simulink model "Rull_tunet_vs_ikketunet"  (R2022a)
settings: Solver=VariableStepAuto  StartTime=0.0  StopTime=25  RelTol=1e-3
values from neighbouring files (symbols this model uses):
  B_r_t = 0.000799434    [Modell_verdier.m]
  C_D = 1.28    [Modell_verdier.m]
  Fb = 226    [Modell_verdier.m]
  g = 9.81    [Modell_verdier.m]
  I_rull = 1.28294    [Modell_verdier.m]
  phi_motor_rull = deg2rad(90-61.7)    [Modell_verdier.m]
  r_Fb = 0.036    [Modell_verdier.m]
  r_motor_rull = 0.277    [Modell_verdier.m]
  tetthet_vann = 1000    [Modell_verdier.m]
libraries: simulink_extras x8, spsFirstOrderFilterLib x2
settings Model: Creator=andre  LastModifiedBy=andre

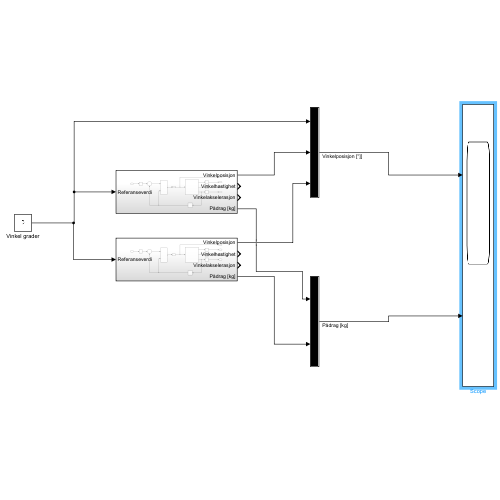
[thumbnail: Simulink's stored preview of the top-level diagram]
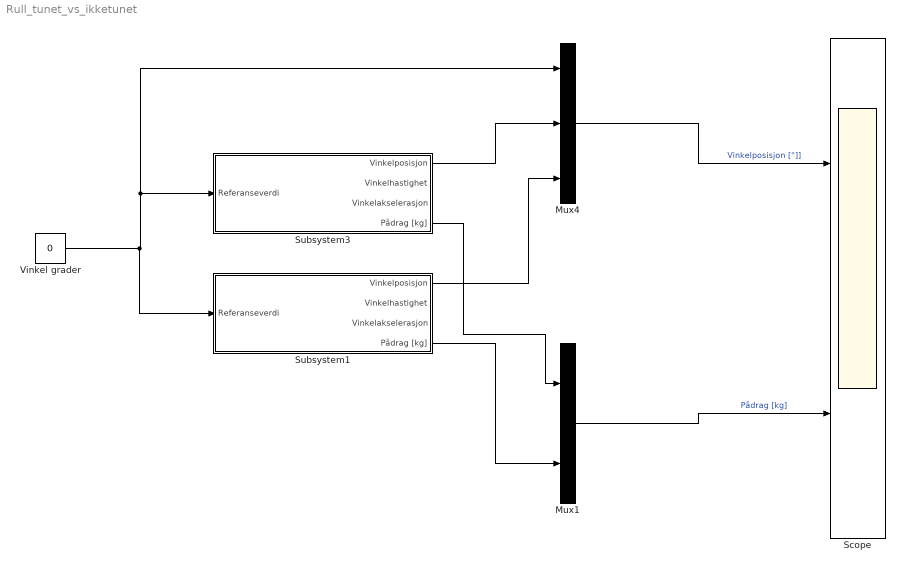
== system Rull_tunet_vs_ikketunet ==
  Mux1 : Mux  Inputs=2
  Mux4 : Mux  Inputs=3
  Scope : Scope  NumInputPorts=2
  Subsystem1 : Subsystem
  Subsystem3 : Subsystem
  Vinkel grader : Constant  Value=0
  wires:
  Vinkel grader/1 -> Subsystem1/1(Referanseverdi), Mux4/1, Subsystem3/1(Referanseverdi)
  Subsystem3/1(Vinkelposisjon) -> Mux4/2
  Subsystem1/1(Vinkelposisjon) -> Mux4/3
  Subsystem1/4(Pådrag [kg]) -> Mux1/2
  Subsystem3/4(Pådrag [kg]) -> Mux1/1
  Mux4/1 -> Scope/1  "Vinkelposisjon [°]]"
  Mux1/1 -> Scope/2  "Pådrag [kg]"

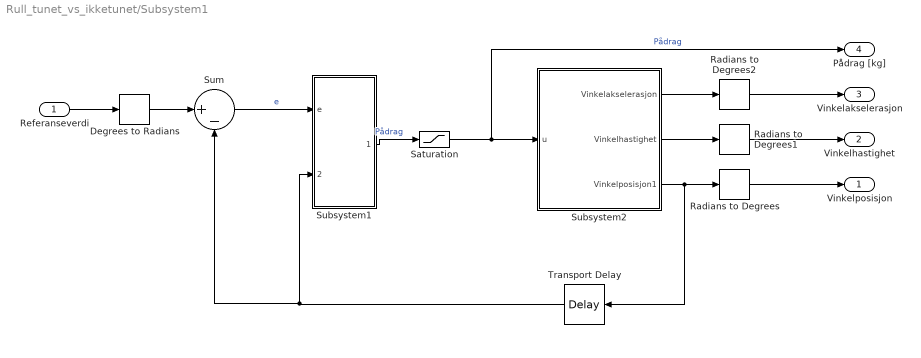
== system Rull_tunet_vs_ikketunet/Subsystem1 ==
  Referanseverdi : Inport
  Degrees to Radians : simulink_extras/Transformations/Degrees to Radians
  Radians to Degrees : simulink_extras/Transformations/Radians to Degrees
  Radians to Degrees1 : simulink_extras/Transformations/Radians to Degrees
  Radians to Degrees2 : simulink_extras/Transformations/Radians to Degrees
  Saturation : Saturate  UpperLimit=2.8  LowerLimit=-2.8
  Subsystem1 : Subsystem
  Subsystem2 : Subsystem
  Sum : Sum  Inputs=|+-
  Transport Delay : TransportDelay  DelayTime=0.2
  Vinkelposisjon : Outport
  Vinkelhastighet : Outport  Port=2
  Vinkelakselerasjon : Outport  Port=3
  Pådrag [kg] : Outport  Port=4
  wires:
  Subsystem2/1(" Vinkelakselerasjon") -> Radians to Degrees2/1
  Sum/1 -> Subsystem1/1(e)  "e"
  Subsystem2/3(Vinkelposisjon1) -> Transport Delay/1, Radians to Degrees/1
  Radians to Degrees/1 -> Vinkelposisjon/1
  Referanseverdi/1 -> Degrees to Radians/1
  Transport Delay/1 -> Sum/2, Subsystem1/2(y_sensor)
  Degrees to Radians/1 -> Sum/1
  Radians to Degrees1/1 -> Vinkelhastighet/1
  Subsystem2/2(" Vinkelhastighet") -> Radians to Degrees1/1
  Saturation/1 -> Pådrag [kg]/1, Subsystem2/1(u)  "Pådrag"
  Subsystem1/1(Pådrag) -> Saturation/1  "Pådrag"
  Radians to Degrees2/1 -> Vinkelakselerasjon/1

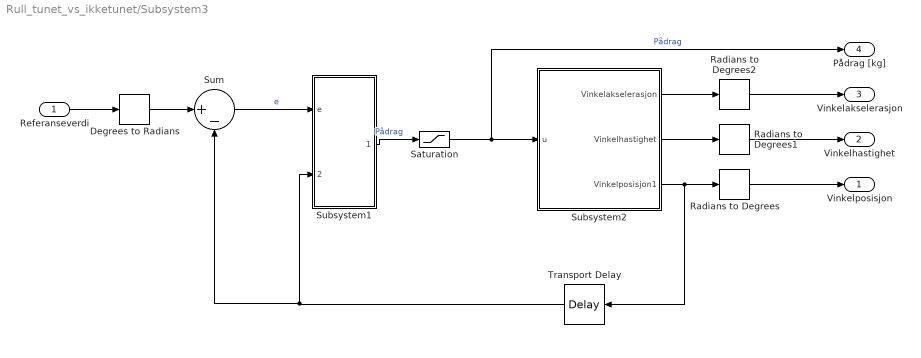
== system Rull_tunet_vs_ikketunet/Subsystem3 ==
  Referanseverdi : Inport
  Degrees to Radians : simulink_extras/Transformations/Degrees to Radians
  Radians to Degrees : simulink_extras/Transformations/Radians to Degrees
  Radians to Degrees1 : simulink_extras/Transformations/Radians to Degrees
  Radians to Degrees2 : simulink_extras/Transformations/Radians to Degrees
  Saturation : Saturate  UpperLimit=2.8  LowerLimit=-2.8
  Subsystem1 : Subsystem
  Subsystem2 : Subsystem
  Sum : Sum  Inputs=|+-
  Transport Delay : TransportDelay  DelayTime=0.2
  Vinkelposisjon : Outport
  Vinkelhastighet : Outport  Port=2
  Vinkelakselerasjon : Outport  Port=3
  Pådrag [kg] : Outport  Port=4
  wires:
  Subsystem2/1(" Vinkelakselerasjon") -> Radians to Degrees2/1
  Sum/1 -> Subsystem1/1(e)  "e"
  Subsystem2/3(Vinkelposisjon1) -> Transport Delay/1, Radians to Degrees/1
  Radians to Degrees/1 -> Vinkelposisjon/1
  Referanseverdi/1 -> Degrees to Radians/1
  Transport Delay/1 -> Sum/2, Subsystem1/2(y_sensor)
  Degrees to Radians/1 -> Sum/1
  Radians to Degrees1/1 -> Vinkelhastighet/1
  Subsystem2/2(" Vinkelhastighet") -> Radians to Degrees1/1
  Saturation/1 -> Pådrag [kg]/1, Subsystem2/1(u)  "Pådrag"
  Subsystem1/1(Pådrag) -> Saturation/1  "Pådrag"
  Radians to Degrees2/1 -> Vinkelakselerasjon/1

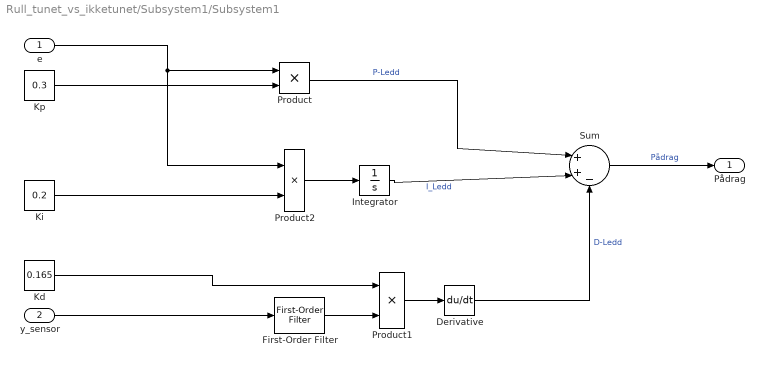
== system Rull_tunet_vs_ikketunet/Subsystem1/Subsystem1 ==
  e : Inport
  y_sensor : Inport  Port=2
  Derivative : Derivative
  First-Order Filter : spsFirstOrderFilterLib/First-Order Filter  FilterType=Lowpass  Tc=(1.5/3.8)*0.05  Ts=0  Initialize=on  Vac_Init=[0, 0, 60]  Vdc_Init=0  PlotResponse=off  FreqRange="[0,  200,  1]"
  Integrator : Integrator  LimitOutput=on  UpperSaturationLimit=0.3  LowerSaturationLimit=-0.3
  Kd : Constant  Value=0.165
  Ki : Constant  Value=0.2
  Kp : Constant  Value=0.3
  Product : Product
  Product1 : Product
  Product2 : Product
  Sum : Sum  Inputs=|++-
  Pådrag : Outport
  wires:
  Product2/1 -> Integrator/1
  Kp/1 -> Product/2
  Product/1 -> Sum/1  "P-Ledd"
  y_sensor/1 -> First-Order Filter/1
  Kd/1 -> Product1/1
  e/1 -> Product/1, Product2/1
  Ki/1 -> Product2/2
  First-Order Filter/1 -> Product1/2
  Integrator/1 -> Sum/2  "I_Ledd"
  Sum/1 -> Pådrag/1  "Pådrag"
  Product1/1 -> Derivative/1
  Derivative/1 -> Sum/3  "D-Ledd"

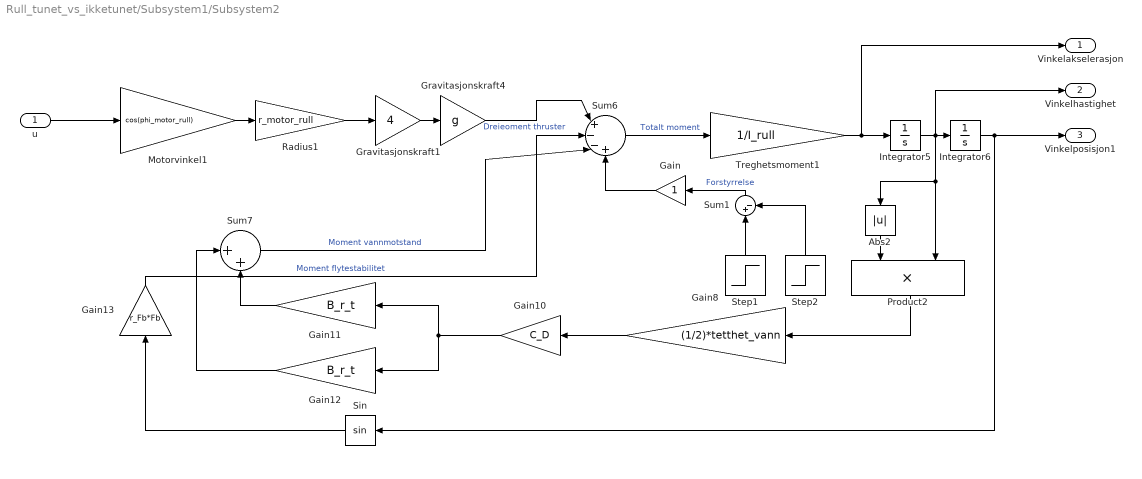
== system Rull_tunet_vs_ikketunet/Subsystem1/Subsystem2 ==
  u : Inport
  Abs2 : Abs  SaturateOnIntegerOverflow=off
  Gain : Gain
  Gain10 : Gain  Gain=C_D
  Gain11 : Gain  Gain=B_r_t
  Gain12 : Gain  Gain=B_r_t
  Gain13 : Gain  Gain=r_Fb*Fb
  Gain8 : Gain  Gain=(1/2)*tetthet_vann
  Gravitasjonskraft1 : Gain  Gain=4
  Gravitasjonskraft4 : Gain  Gain=g
  Integrator5 : Integrator
  Integrator6 : Integrator
  Motorvinkel1 : Gain  Gain=cos(phi_motor_rull)
  Product2 : Product
  Radius1 : Gain  Gain=r_motor_rull
  Sin : Trigonometry
  Step1 : Step  Time=7  After=5  SampleTime=0
  Step2 : Step  Time=10  After=0  SampleTime=0
  Sum1 : Sum  Inputs=|+-
  Sum6 : Sum  Inputs=|+--+
  Sum7 : Sum  Inputs=|++
  Treghetsmoment1 : Gain  Gain=1/I_rull
  " Vinkelakselerasjon" : Outport
  " Vinkelhastighet" : Outport  Port=2
  Vinkelposisjon1 : Outport  Port=3
  wires:
  Integrator6/1 -> Vinkelposisjon1/1, Sin/1
  Motorvinkel1/1 -> Radius1/1
  Gain8/1 -> Gain10/1
  Integrator5/1 -> " Vinkelhastighet"/1, Abs2/1, Product2/2, Integrator6/1
  Treghetsmoment1/1 -> " Vinkelakselerasjon"/1, Integrator5/1
  Gain11/1 -> Sum7/2
  Sum7/1 -> Sum6/3  "Moment vannmotstand"
  Gravitasjonskraft4/1 -> Sum6/1  "Dreieoment thruster"
  Sum6/1 -> Treghetsmoment1/1  "Totalt moment"
  Gain10/1 -> Gain12/1, Gain11/1
  Sin/1 -> Gain13/1
  Product2/1 -> Gain8/1
  Radius1/1 -> Gravitasjonskraft1/1
  Gain12/1 -> Sum7/1
  Gravitasjonskraft1/1 -> Gravitasjonskraft4/1
  Abs2/1 -> Product2/1
  Gain13/1 -> Sum6/2  "Moment flytestabilitet"
  u/1 -> Motorvinkel1/1
  Gain/1 -> Sum6/4
  Sum1/1 -> Gain/1  "Forstyrrelse"
  Step1/1 -> Sum1/1
  Step2/1 -> Sum1/2

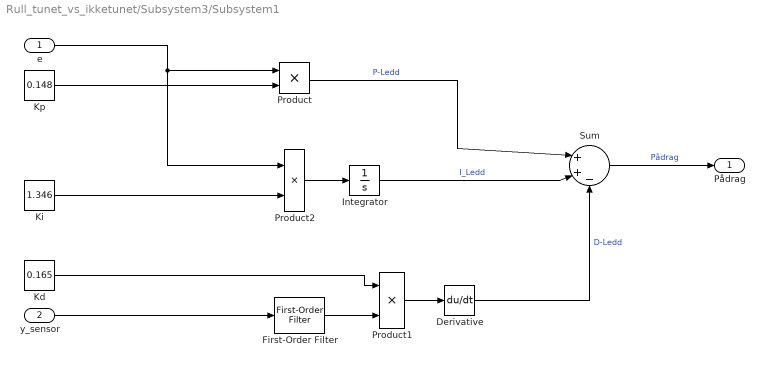
== system Rull_tunet_vs_ikketunet/Subsystem3/Subsystem1 ==
  e : Inport
  y_sensor : Inport  Port=2
  Derivative : Derivative
  First-Order Filter : spsFirstOrderFilterLib/First-Order Filter  FilterType=Lowpass  Tc=(1.5/3.8)*0.05  Ts=0  Initialize=on  Vac_Init=[0, 0, 60]  Vdc_Init=0  PlotResponse=off  FreqRange="[0,  200,  1]"
  Integrator : Integrator  LimitOutput=on  UpperSaturationLimit=0.3  LowerSaturationLimit=-0.3
  Kd : Constant  Value=0.165
  Ki : Constant  Value=1.346
  Kp : Constant  Value=0.148
  Product : Product
  Product1 : Product
  Product2 : Product
  Sum : Sum  Inputs=|++-
  Pådrag : Outport
  wires:
  Product2/1 -> Integrator/1
  Kp/1 -> Product/2
  Product/1 -> Sum/1  "P-Ledd"
  y_sensor/1 -> First-Order Filter/1
  Kd/1 -> Product1/1
  e/1 -> Product/1, Product2/1
  Ki/1 -> Product2/2
  First-Order Filter/1 -> Product1/2
  Integrator/1 -> Sum/2  "I_Ledd"
  Sum/1 -> Pådrag/1  "Pådrag"
  Product1/1 -> Derivative/1
  Derivative/1 -> Sum/3  "D-Ledd"

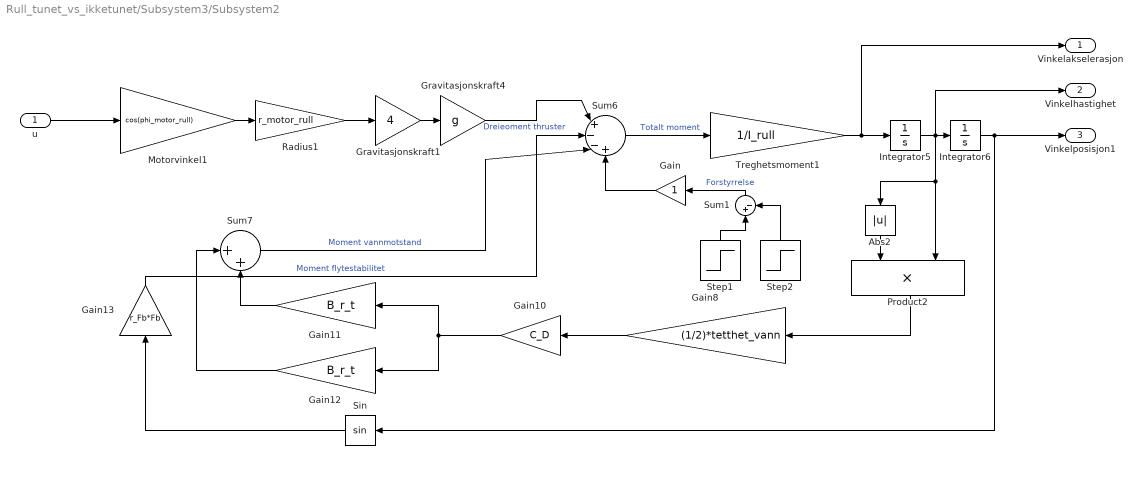
== system Rull_tunet_vs_ikketunet/Subsystem3/Subsystem2 ==
  u : Inport
  Abs2 : Abs  SaturateOnIntegerOverflow=off
  Gain : Gain
  Gain10 : Gain  Gain=C_D
  Gain11 : Gain  Gain=B_r_t
  Gain12 : Gain  Gain=B_r_t
  Gain13 : Gain  Gain=r_Fb*Fb
  Gain8 : Gain  Gain=(1/2)*tetthet_vann
  Gravitasjonskraft1 : Gain  Gain=4
  Gravitasjonskraft4 : Gain  Gain=g
  Integrator5 : Integrator
  Integrator6 : Integrator  InitialCondition=2*pi/9
  Motorvinkel1 : Gain  Gain=cos(phi_motor_rull)
  Product2 : Product
  Radius1 : Gain  Gain=r_motor_rull
  Sin : Trigonometry
  Step1 : Step  Time=7  After=5  SampleTime=0
  Step2 : Step  Time=10  After=5  SampleTime=0
  Sum1 : Sum  Inputs=|+-
  Sum6 : Sum  Inputs=|+--+
  Sum7 : Sum  Inputs=|++
  Treghetsmoment1 : Gain  Gain=1/I_rull
  " Vinkelakselerasjon" : Outport
  " Vinkelhastighet" : Outport  Port=2
  Vinkelposisjon1 : Outport  Port=3
  wires:
  Integrator6/1 -> Vinkelposisjon1/1, Sin/1
  Motorvinkel1/1 -> Radius1/1
  Gain8/1 -> Gain10/1
  Integrator5/1 -> " Vinkelhastighet"/1, Abs2/1, Product2/2, Integrator6/1
  Treghetsmoment1/1 -> " Vinkelakselerasjon"/1, Integrator5/1
  Gain11/1 -> Sum7/2
  Sum7/1 -> Sum6/3  "Moment vannmotstand"
  Gravitasjonskraft4/1 -> Sum6/1  "Dreieoment thruster"
  Sum6/1 -> Treghetsmoment1/1  "Totalt moment"
  Gain10/1 -> Gain12/1, Gain11/1
  Sin/1 -> Gain13/1
  Product2/1 -> Gain8/1
  Radius1/1 -> Gravitasjonskraft1/1
  Gain12/1 -> Sum7/1
  Gravitasjonskraft1/1 -> Gravitasjonskraft4/1
  Abs2/1 -> Product2/1
  Gain13/1 -> Sum6/2  "Moment flytestabilitet"
  u/1 -> Motorvinkel1/1
  Gain/1 -> Sum6/4
  Step1/1 -> Sum1/1
  Sum1/1 -> Gain/1  "Forstyrrelse"
  Step2/1 -> Sum1/2
